simulink model "DP2Model"  (R2019a)
settings: Solver=VariableStepAuto  StartTime=0.0  StopTime=2  FixedStep=0.0001  MaxStep=0.001  RelTol=1e-3
values from neighbouring files (symbols this model uses):
  A = 1/JT *[zeros(2,2),JT*eye(2,2);     0 ,1/4 * mp^2 *Lp^2*Lr*g, -(Jp + 1/4 *mp*Lp^2)*Dr, -1/2*mp*Lr*Lp*Dp;     0,1/2 *mp*Lp*g*(Jr + mp*Lr^2),-1/2*mp*Lp*Lr*Dr, -(Jr +mp*Lr^2)*Dp]    [dp2script.m]    (also in jacobA.m = [0,0,1,0;0,0,0,1;0,Lp.*mp.*Rm.^(-1).*((-4).*Lp.^2.*Lr.^2.*mp)
  B = ng*nm*Kg*Kt /Rm *B    [dp2script.m]    (also in jacobA.m = [0;0;4.*Kg.*Kt.*(4.*Jp+Lp.^2.*mp).*n.*Rm.^(-1).*((-4).*Lp.^2; nonLinear.m = [(tau-Dr*dtheta); -Dp*dalpha])
  C = eye(2,4)    [dp2script.m]    (also in nonLinear.m = [A3, A4;B3,0])
  g = 9.81    [dp2script.m]    (also in jacobA.m; nonLinear.m)
  Jp = 0.0012    [dp2script.m]    (also in jacobA.m; nonLinear.m)
  K = place(A,B,p)    [dp2script.m]    (also in placeA.m = Bv(:,1:m) * K)
  Kg = 70    [dp2script.m]    (also in jacobA.m; nonLinear.m)
  km = 7.68e-3    (= 0.00768)    [dp2script.m]    (also in jacobA.m; nonLinear.m)
  Kt = 7.68e-3    (= 0.00768)    [dp2script.m]    (also in jacobA.m; nonLinear.m)
  Lp = 0.129    [dp2script.m]    (also in jacobA.m; nonLinear.m)
  Lr = 0.085    [dp2script.m]    (also in jacobA.m; nonLinear.m)
  mp = 0.127    [dp2script.m]    (also in jacobA.m; nonLinear.m)
  mr = 0.257    [dp2script.m]    (also in jacobA.m; nonLinear.m)
  n = ng*nm    (= 0.621)    [dp2script.m]    (also in jacobA.m; nonLinear.m)
  Rm = 8.40    (= 8.4)    [dp2script.m]    (also in jacobA.m; nonLinear.m)
libraries: simulink x2
settings Model: Creator=Ankith A Das  LastModifiedBy=Ankith A Das

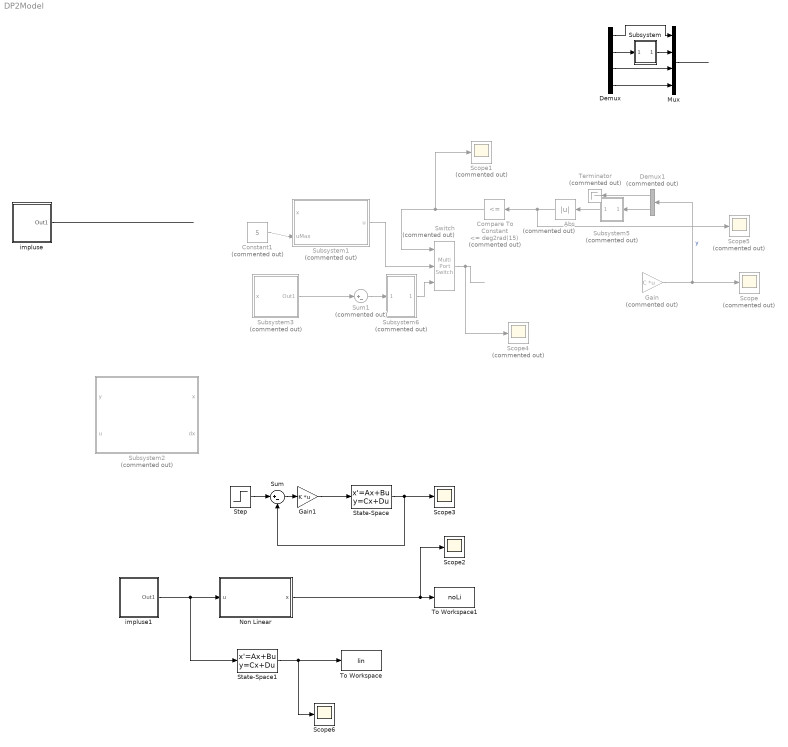
== system DP2Model ==
  Abs : Abs  Commented=on
  Compare To Constant : simulink/Logic and Bit Operations/Compare To Constant  Commented=on  relop=<=  const=deg2rad(15)  OutDataTypeStr=uint8
  Constant1 : Constant  Commented=on  Value=5
  Demux : Demux
  Demux1 : Demux  Commented=on  Outputs=2
  Gain : Gain  Commented=on  Gain=C  Multiplication=Matrix(K*u)
  Gain1 : Gain  Gain=K  Multiplication=Matrix(K*u)
  Mux : Mux
  Non Linear : Subsystem
  Scope{,1,4..5} (4 alike) : Scope  Commented=on
  Scope2 : Scope
  Scope3 : Scope
  Scope6 : Scope
  State-Space : StateSpace  A=A  B=B  C=eye(4)  D=zeros(4,1)  InitialCondition=[0.05,0,0,0]'
  State-Space1 : StateSpace  A=A  B=B  C=eye(4)  D=zeros(4,1)  InitialCondition=[0,0,0,0]'
  Step : Step  Before=[0,0,0,0]'  After=[deg2rad(10),0,0,0]'  SampleTime=0
  Subsystem : Subsystem
  Subsystem1 : Subsystem  Commented=on
  Subsystem2 : Subsystem  Commented=on
  Subsystem3 : Subsystem  Commented=on
  Subsystem5 : Subsystem  Commented=on
  Subsystem6 : Subsystem  Commented=on
  Sum : Sum  Inputs=|+-
  Sum1 : Sum  Commented=on  Inputs=|+-
  Switch : MultiPortSwitch  Commented=on  DataPortOrder=Zero-based contiguous  Inputs=2  zeroidx=on
  Terminator : Terminator  Commented=on
  To Workspace : ToWorkspace  VariableName=lin  SaveFormat=Structure With Time  SampleTime=-1
  To Workspace1 : ToWorkspace  VariableName=noLi  SaveFormat=Structure With Time  SampleTime=-1
  impluse : Subsystem
  impluse1 : Subsystem
  wires:
  State-Space/1 -> Sum/2, Scope3/1
  Gain/1 -> Demux1/1, Scope/1  "y"
  Mux/1 -> ?
  Demux1/2 -> Subsystem5/1(In1)
  Subsystem/1(Out1) -> Mux/2
  Demux/4 -> Mux/4
  Demux/3 -> Mux/3
  Demux/2 -> Subsystem/1(In1)
  Demux/1 -> Mux/1
  Sum/1 -> Gain1/1
  Step/1 -> Sum/1
  Gain1/1 -> State-Space/1
  impluse/1(Out1) -> ?
  Abs/1 -> Scope5/1, Compare To Constant/1
  Demux1/1 -> Terminator/1
  Constant1/1 -> Subsystem1/2(uMax)
  Subsystem1/1(u) -> Switch/2
  Subsystem5/1(Out1) -> Abs/1
  Subsystem3/1(Out1) -> Sum1/1
  ? -> Gain/1, Sum1/2, Subsystem1/1(x), Subsystem3/1(x)
  Switch/1 -> Scope4/1
  Sum1/1 -> Subsystem6/1(In1)
  Subsystem6/1(Out1) -> Switch/3
  Compare To Constant/1 -> Scope1/1, Switch/1
  impluse1/1(Out1) -> State-Space1/1, Non Linear/1(u)
  Non Linear/1(x) -> Scope2/1, To Workspace1/1
  State-Space1/1 -> Scope6/1, To Workspace/1

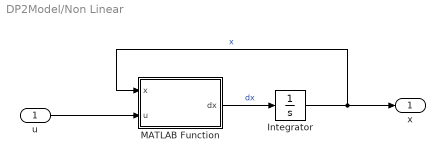
== system DP2Model/Non Linear ==
  u : Inport
  Integrator : Integrator  InitialCondition=[0,0,0,0]'
  MATLAB Function : MATLAB Function  TreatAsAtomicUnit=on
  x : Outport
  wires:
  Integrator/1 -> x/1, MATLAB Function/1(x)  "x"
  u/1 -> MATLAB Function/2(u)
  MATLAB Function/1(dx) -> Integrator/1  "dx"

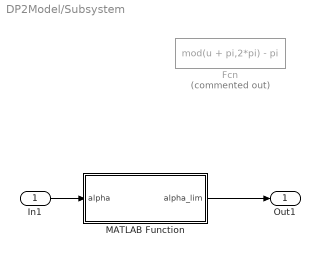
== system DP2Model/Subsystem ==
  In1 : Inport
  Fcn : Fcn  Commented=on  Expr=mod(u + pi,2*pi) - pi
  MATLAB Function : MATLAB Function  TreatAsAtomicUnit=on
  Out1 : Outport
  wires:
  In1/1 -> MATLAB Function/1(alpha)
  MATLAB Function/1(alpha_lim) -> Out1/1

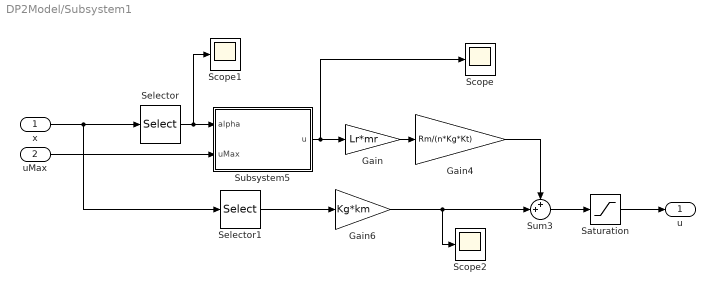
== system DP2Model/Subsystem1 ==
  x : Inport
  uMax : Inport  Port=2
  Gain : Gain  Gain=Lr*mr
  Gain4 : Gain  Gain=Rm/(n*Kg*Kt)
  Gain6 : Gain  Gain=Kg*km
  Saturation : Saturate  UpperLimit=5  LowerLimit=-5
  Scope : Scope
  Scope1 : Scope
  Scope2 : Scope
  Selector : Selector  InputPortWidth=4  IndexOptions=Index vector (dialog)  Indices=[2 4]  OutputSizes=1
  Selector1 : Selector  InputPortWidth=4  IndexOptions=Index vector (dialog)  Indices=[3]  OutputSizes=1
  Subsystem5 : Subsystem
  Sum3 : Sum  Inputs=++|
  u : Outport
  wires:
  Gain6/1 -> Scope2/1, Sum3/2
  Subsystem5/1(u) -> Gain/1, Scope/1
  Selector/1 -> Scope1/1, Subsystem5/1(alpha)
  x/1 -> Selector1/1, Selector/1
  Gain/1 -> Gain4/1
  Gain4/1 -> Sum3/1
  uMax/1 -> Subsystem5/2("uMax ")
  Selector1/1 -> Gain6/1
  Sum3/1 -> Saturation/1
  Saturation/1 -> u/1

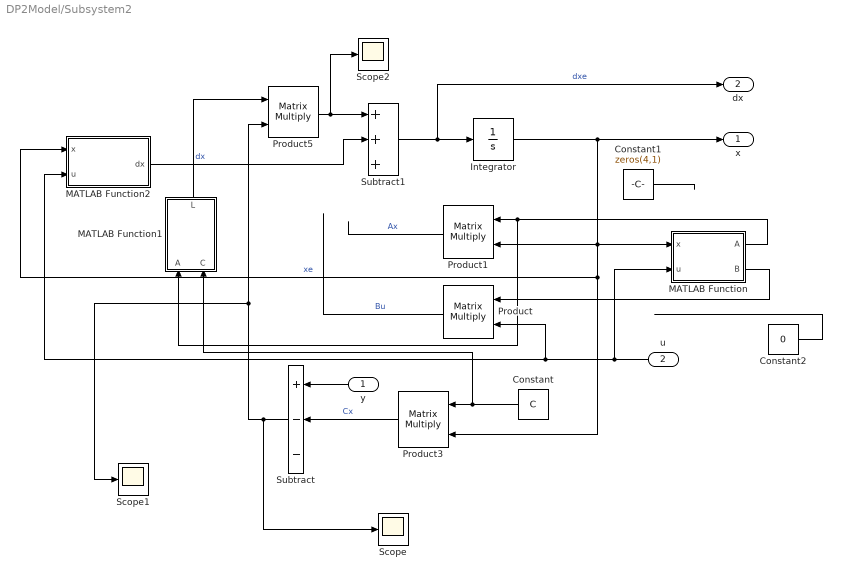
== system DP2Model/Subsystem2 ==
  y : Inport
  u : Inport  Port=2
  Constant : Constant  Value=C
  Constant1 : Constant  Value=zeros(4,1)
  Constant2 : Constant  Value=0
  Integrator : Integrator  InitialCondition=rand(4,1)*5
  MATLAB Function : MATLAB Function  TreatAsAtomicUnit=on
  MATLAB Function1 : MATLAB Function  TreatAsAtomicUnit=on
  MATLAB Function2 : MATLAB Function  TreatAsAtomicUnit=on
  Product{,1,3,5} (4 alike) : Product  SCDEnableBlockLinearizationSpecification=on  Multiplication=Matrix(*)
  Scope : Scope
  Scope1 : Scope
  Scope2 : Scope
  Subtract : Sum  Inputs=+--
  Subtract1 : Sum  Inputs=+++
  x : Outport
  dx : Outport  Port=2
  wires:
  Subtract1/1 -> dx/1, Integrator/1  "dxe"
  y/1 -> Subtract/1
  MATLAB Function1/1(L) -> Product5/1
  Subtract/1 -> Scope1/1, Product5/2, Scope/1
  Product5/1 -> Scope2/1, Subtract1/1
  Product1/1 -> ?  "Ax"
  Constant/1 -> MATLAB Function1/2(C), Product3/1
  Product/1 -> ?  "Bu"
  Product3/1 -> Subtract/2  "Cx"
  Integrator/1 -> x/1, MATLAB Function/1(x), Product1/2, Product3/2, MATLAB Function2/1(x)  "xe"
  u/1 -> MATLAB Function2/2(u), Product/2, MATLAB Function/2(u)
  MATLAB Function/1(A) -> Product1/1, MATLAB Function1/1(A)
  MATLAB Function/2(B) -> Product/1
  Constant1/1 -> ?
  Constant2/1 -> ?
  MATLAB Function2/1(dx) -> Subtract1/2  "dx"

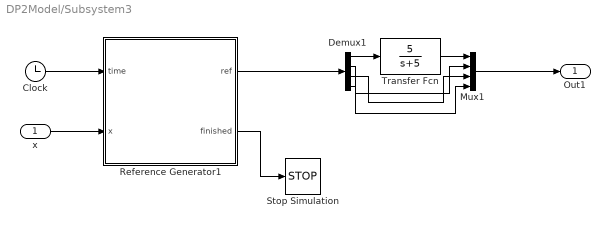
== system DP2Model/Subsystem3 ==
  x : Inport
  Clock : Clock
  Demux1 : Demux
  Mux1 : Mux
  Reference Generator1 : MATLAB Function  TreatAsAtomicUnit=on  SystemSampleTime=0.002
  Stop Simulation : Stop
  Transfer Fcn : TransferFcn  Numerator=[5]  Denominator=[1 5]
  Out1 : Outport
  wires:
  Demux1/1 -> Transfer Fcn/1
  Mux1/1 -> Out1/1
  Demux1/4 -> Mux1/4
  Demux1/3 -> Mux1/3
  Demux1/2 -> Mux1/2
  x/1 -> Reference Generator1/2(x)
  Reference Generator1/1(ref) -> Demux1/1
  Reference Generator1/2(finished) -> Stop Simulation/1
  Transfer Fcn/1 -> Mux1/1
  Clock/1 -> Reference Generator1/1(time)

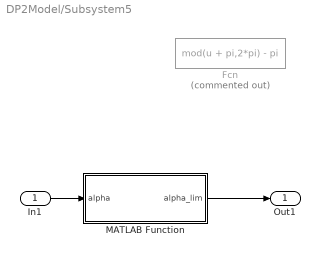
== system DP2Model/Subsystem5 ==
  In1 : Inport
  Fcn : Fcn  Commented=on  Expr=mod(u + pi,2*pi) - pi
  MATLAB Function : MATLAB Function  TreatAsAtomicUnit=on
  Out1 : Outport
  wires:
  In1/1 -> MATLAB Function/1(alpha)
  MATLAB Function/1(alpha_lim) -> Out1/1

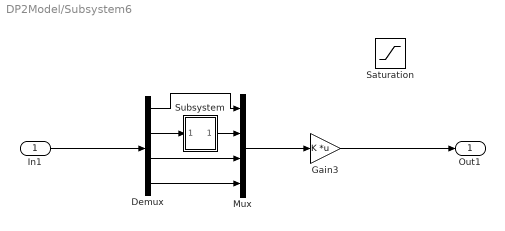
== system DP2Model/Subsystem6 ==
  In1 : Inport
  Demux : Demux
  Gain3 : Gain  Gain=K  Multiplication=Matrix(K*u)
  Mux : Mux
  Saturation : Saturate  UpperLimit=6  LowerLimit=-6
  Subsystem : Subsystem
  Out1 : Outport
  wires:
  In1/1 -> Demux/1
  Demux/1 -> Mux/1
  Demux/4 -> Mux/4
  Demux/2 -> Subsystem/1(In1)
  Demux/3 -> Mux/3
  Subsystem/1(Out1) -> Mux/2
  Mux/1 -> Gain3/1
  Gain3/1 -> Out1/1

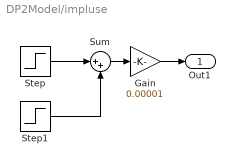
== system DP2Model/impluse ==
  Gain : Gain  Gain=0.00001
  Step : Step  Time=0  SampleTime=0
  Step1 : Step  After=-1  SampleTime=0
  Sum : Sum  Inputs=|++
  Out1 : Outport
  wires:
  Step/1 -> Sum/1
  Step1/1 -> Sum/2
  Sum/1 -> Gain/1
  Gain/1 -> Out1/1

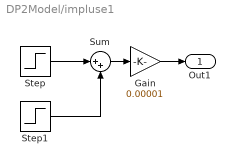
== system DP2Model/impluse1 ==
  Gain : Gain  Gain=0.00001
  Step : Step  Time=0  SampleTime=0
  Step1 : Step  After=-1  SampleTime=0
  Sum : Sum  Inputs=|++
  Out1 : Outport
  wires:
  Step/1 -> Sum/1
  Step1/1 -> Sum/2
  Sum/1 -> Gain/1
  Gain/1 -> Out1/1

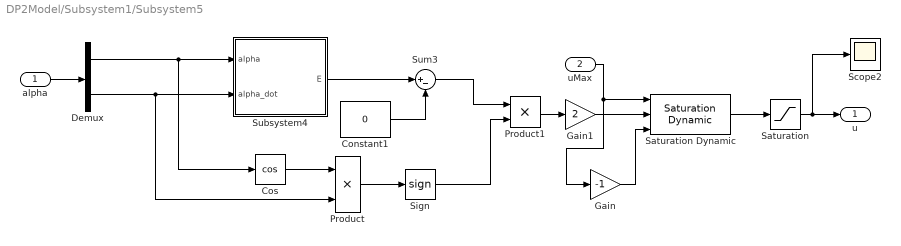
== system DP2Model/Subsystem1/Subsystem5 ==
  alpha : Inport
  "uMax " : Inport  Port=2
  Constant1 : Constant  Value=0
  Cos : Trigonometry  Operator=cos
  Demux : Demux  Outputs=2
  Gain : Gain  Gain=-1
  Gain1 : Gain  Gain=2
  Product : Product
  Product1 : Product
  Saturation : Saturate  UpperLimit=10  LowerLimit=-10
  Saturation Dynamic : simulink/Discontinuities/Saturation Dynamic  OutMin=[]  OutMax=[]  OutDataTypeStr=Inherit: Same as second input  OutDataType=fixdt(1, 16)  OutScaling=2^-10  DoSatur=off
  Scope2 : Scope
  Sign : Signum  ZeroCross=off
  Subsystem4 : Subsystem
  Sum3 : Sum  Inputs=|+-
  u : Outport
  wires:
  Demux/1 -> Cos/1, Subsystem4/1(alpha)
  Subsystem4/1(E) -> Sum3/1
  Demux/2 -> Product/2, Subsystem4/2(alpha_dot)
  Cos/1 -> Product/1
  Product/1 -> Sign/1
  Constant1/1 -> Sum3/2
  Product1/1 -> Gain1/1
  "uMax "/1 -> Saturation Dynamic/1, Gain/1
  Gain/1 -> Saturation Dynamic/3
  Saturation Dynamic/1 -> Saturation/1
  alpha/1 -> Demux/1
  Gain1/1 -> Saturation Dynamic/2
  Saturation/1 -> Scope2/1, u/1
  Sum3/1 -> Product1/1
  Sign/1 -> Product1/2

== system DP2Model/Subsystem6/Subsystem ==
  In1 : Inport
  Fcn : Fcn  Commented=on  Expr=mod(u + pi,2*pi) - pi
  MATLAB Function : MATLAB Function  TreatAsAtomicUnit=on
  Out1 : Outport
  wires:
  In1/1 -> MATLAB Function/1(alpha)
  MATLAB Function/1(alpha_lim) -> Out1/1

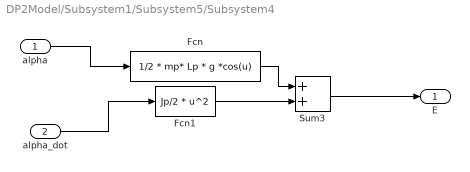
== system DP2Model/Subsystem1/Subsystem5/Subsystem4 ==
  alpha : Inport
  alpha_dot : Inport  Port=2
  Fcn : Fcn  Expr=1/2 * mp* Lp * g *cos(u)
  Fcn1 : Fcn  Expr=Jp/2 * u^2
  Sum3 : Sum
  E : Outport
  wires:
  alpha/1 -> Fcn/1
  Sum3/1 -> E/1
  Fcn/1 -> Sum3/1
  Fcn1/1 -> Sum3/2
  alpha_dot/1 -> Fcn1/1

== matlab function DP2Model/Subsystem2/MATLAB Function ==
  data: x input; u input; A output; B output
function [A,B] = fcn(x,u)
    [A,B] = jacobA(x,u);
    
    %A = zeros(4,4);
    %B = zeros(4,1);
end

== matlab function DP2Model/Non Linear/MATLAB Function ==
  data: x input; u input; dx output
function dx = fullSystem(x,u)
    dx = nonLinear(x,u);
end

== matlab function DP2Model/Subsystem2/MATLAB Function1 ==
  data: A input; L output; C input
function L = fcn(A,C)
   L = placeA(A',C',[-2,-91,-95,-90]).';
end

== matlab function DP2Model/Subsystem2/MATLAB Function2 ==
  data: x input; u input; dx output
function dx = fullSystem(x,u)
    dx = nonLinear(x,u);
end

== matlab function DP2Model/Subsystem3/Reference Generator1 ==
  data: time input; x input size=4; ref output; finished output
function [ref, finished] = REFGEN(time, x)


persistent n 

persistent goodSteps 
persistent done
persistent recTime

if(isempty(n))
    n = 1; % start at first waypoint
    done = false;
end
if(isempty(goodSteps))
    goodSteps = 1;
end
if(isempty(recTime))
    recTime = -1; % start at first waypoint
end
    ref = zeros(4,1);
    x(2) = mod(x(2) + pi,2*pi)-pi;
    % Local variables
    waypoints = [30; -60; 45; -30]*pi/180; % reference waypoints
    posTolArm = 1*pi/180; % [rad] position tolerance
    posTolPend = posTolArm;
    velTolArm = 0.1; % [rad/s] velocity tolerance
    velTolPend = 0.1; % [rad/s] basically KF tolerance.

    if (abs(waypoints(n)-x(1)) <= posTolArm) && (abs(x(2)) <= posTolPend) && (abs(x(3)) <= velTolArm) && (abs(x(4)) <= velTolPend) % q1 and q2 stationary
        goodSteps = goodSteps + 1; % increment count if everything satisifed this timestep
        if recTime == -1
            recTime = time;
        end
    else
        goodSteps = 1; % reset if tolerances breached
        recTime = -1;
    end

    rst = false;
    %% detect successful completion of waypoint
    holdTime = 3;
    if time - recTime >= holdTime && recTime ~= -1
        rst = true;
        n = n + 1;
        if n > length(waypoints)
            done = true;
        end
        recTime = -1;
    end
%% Output reference
if(~done)
    ref(1) = waypoints(n);
    finished = done;
else
    ref(1) = waypoints(end);
    finished = done;
end

== matlab function DP2Model/Subsystem/MATLAB Function ==
  data: alpha input; alpha_lim output
function alpha_lim = fcn(alpha)
    alpha_lim = mod(alpha + pi,2*pi)-pi;
end

== matlab function DP2Model/Subsystem5/MATLAB Function ==
  data: alpha input; alpha_lim output
function alpha_lim = fcn(alpha)
    alpha_lim = mod(alpha + pi,2*pi)-pi;
end

== matlab function DP2Model/Subsystem6/Subsystem/MATLAB Function ==
  data: alpha input; alpha_lim output
function alpha_lim = fcn(alpha)
    alpha_lim = mod(alpha + pi,2*pi)-pi;
end
